simulink model "SR-to-MP_simulation_system"  (R2019a)
settings: Solver=VariableStepAuto  StartTime=0.0  StopTime=720000  RelTol=1e-3
undefined symbols (not defined in the file or in its folder): des
settings Model: Creator=86180  LastModifiedBy=86180

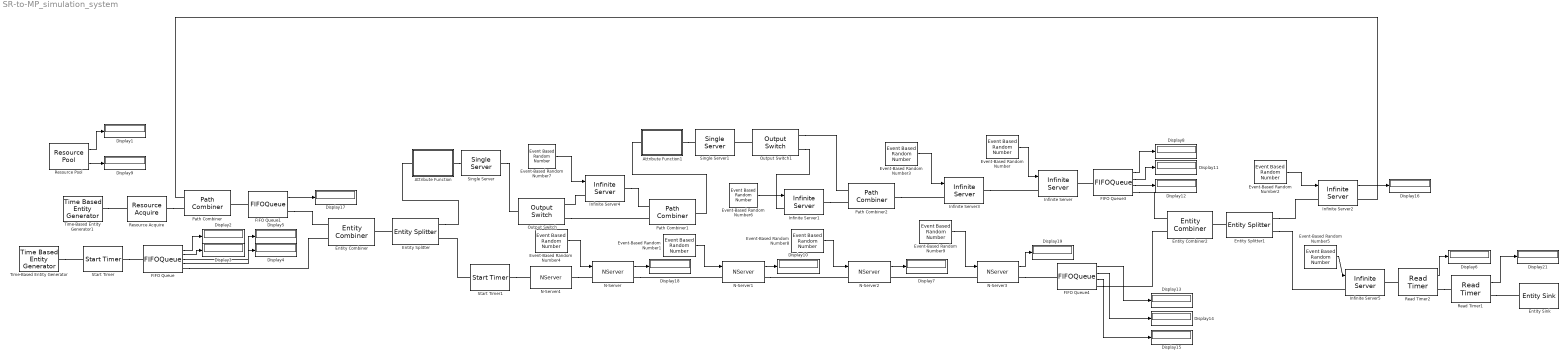
== system SR-to-MP_simulation_system ==
  Attribute Function : Subsystem  LoadFcn=des.afb.attributefunction_support(gcb,'LoadFcn');  StartFcn=des.afb.attributefunction_support(gcb,'StartFcn');  mask(Attribute Function){OutputNamePrefix=out_}
      mask prompts: OutputNamePrefix "Prefix name"
      settings: CopyFcn=des.afb.attributefunction_support(gcb,'CopyFcn');  OpenFcn=des.afb.attributefunction_support(gcb,'OpenFcn');  ErrorFcn=des.afb.error_redirect
      mask Help: slhelp(gcbh)
      mask Display: image(des_iconLoad('attribFunction.jpg'),'center');
  Attribute Function1 : Subsystem  LoadFcn=des.afb.attributefunction_support(gcb,'LoadFcn');  StartFcn=des.afb.attributefunction_support(gcb,'StartFcn');  mask(Attribute Function){OutputNamePrefix=out_}
      mask prompts: OutputNamePrefix "Prefix name"
      settings: CopyFcn=des.afb.attributefunction_support(gcb,'CopyFcn');  OpenFcn=des.afb.attributefunction_support(gcb,'OpenFcn');  ErrorFcn=des.afb.error_redirect
      mask Help: slhelp(gcbh)
      mask Display: image(des_iconLoad('attribFunction.jpg'),'center');
  Display{1..19,21} (20 alike) : Display
  Entity Combiner : EntityCombiner  NumberInputPorts=2
  Entity Combiner2 : EntityCombiner  NumberInputPorts=2
  Entity Sink : EntitySink
  Entity Splitter : EntitySplitter  NumberOutputPorts=2
  Entity Splitter1 : EntitySplitter  NumberOutputPorts=2
  Event-Based Random Number : EventBasedRandomNumber  meanExp=387  meanNorm=315  stdNorm=5  Seed=34425
  Event-Based Random Number1 : EventBasedRandomNumber  meanExp=234  meanNorm=7  stdNorm=38  Seed=3080
  Event-Based Random Number2 : EventBasedRandomNumber  meanExp=10  Seed=58140
  Event-Based Random Number3 : EventBasedRandomNumber  meanExp=10  meanNorm=12  stdNorm=3  Seed=11223
  Event-Based Random Number4 : EventBasedRandomNumber  meanExp=234  meanNorm=7  stdNorm=38  Seed=343
  Event-Based Random Number5 : EventBasedRandomNumber  meanExp=10  Seed=61357
  Event-Based Random Number6 : EventBasedRandomNumber  meanExp=3  meanNorm=12  stdNorm=3  Seed=251
  Event-Based Random Number7 : EventBasedRandomNumber  meanExp=3  meanNorm=12  stdNorm=3  Seed=2512
  Event-Based Random Number8 : EventBasedRandomNumber  meanExp=234  meanNorm=7  stdNorm=38  Seed=3423
  Event-Based Random Number9 : EventBasedRandomNumber  meanExp=234  meanNorm=7  stdNorm=38  Seed=3423
  FIFO Queue : FIFOQueue  Capacity=10000  StatNumberDeparted=on  StatNumberInBlock=on  StatAverageWait=on  StatAverageQueueLength=on
      settings: OutputPortMap=o0,o1,o2,o3
  FIFO Queue1 : FIFOQueue  Capacity=100  StatAverageQueueLength=on
      settings: OutputPortMap=o3
  FIFO Queue3 : FIFOQueue  StatNumberDeparted=on  StatAverageWait=on  StatAverageQueueLength=on
      settings: OutputPortMap=o0,o2,o3
  FIFO Queue4 : FIFOQueue  Capacity=6  StatNumberDeparted=on  StatAverageWait=on  StatAverageQueueLength=on
      settings: OutputPortMap=o0,o2,o3
  Infinite Server{,1,3..5} (5 alike) : InfiniteServer  ServiceTimeFrom=Signal port t
  Infinite Server2 : InfiniteServer  ServiceTimeFrom=Signal port t  StatNumberDeparted=on
  N-Server{,1..3} (4 alike) : NServer  NumberOfServers=6  ServiceTimeFrom=Signal port t  StatUtilization=on
      settings: OutputPortMap=o5
  N-Server4 : NServer  NumberOfServers=10  ServiceTime=0
  Output Switch : OutputSwitch  NumberOutputPorts=2  SwitchingCriterion=From attribute  AttributeName=Attribute
  Output Switch1 : OutputSwitch  NumberOutputPorts=2  SwitchingCriterion=From attribute  AttributeName=Attribute2
  Path Combiner : PathCombiner  NumberInputPorts=2
  Path Combiner1 : PathCombiner  NumberInputPorts=2
  Path Combiner2 : PathCombiner  NumberInputPorts=2
  Read Timer1 : ReadTimer  TimerTag=T2  StatAverageTimeElapsed=on
      settings: OutputPortMap=o3
  Read Timer2 : ReadTimer  StatAverageTimeElapsed=on
      settings: OutputPortMap=o3
  Resource Acquire : ResourceAcquire  ResourceName=robot  Capacity=100  EvaluatedResourceAmount={ 1}
  Resource Pool : ResourcePool  ResourceName=robot  ResourceAmount=18  StatAmountInUse=on  StatUtilization=on
      settings: OutputPortMap=o0,o1
  Single Server : SingleServer  ServiceTime=0
  Single Server1 : SingleServer  ServiceTime=0
  Start Timer : StartTimer  TimerTag=T2  TimerStartedOption=Continue
  Start Timer1 : StartTimer  TimerStartedOption=Continue
  Time-Based Entity Generator : TimeBasedEntityGenerator  Distribution=Exponential  InitialSeed=40859  Mean=3600/60
  Time-Based Entity Generator1 : TimeBasedEntityGenerator  Period=0.00000001  Mean=3600/20
  wires:
  Event-Based Random Number1/1 -> N-Server1/1
  Event-Based Random Number4/1 -> N-Server/1
  Event-Based Random Number2/1 -> Infinite Server2/1
  FIFO Queue4/1 -> Display13/1
  FIFO Queue4/2 -> Display14/1
  Resource Pool/1 -> Display1/1
  Infinite Server2/1 -> Display16/1
  Event-Based Random Number/1 -> Infinite Server/1
  FIFO Queue/4 -> Display4/1
  Event-Based Random Number3/1 -> Infinite Server3/1
  FIFO Queue3/3 -> Display12/1
  FIFO Queue1/1 -> Display17/1
  FIFO Queue/3 -> Display5/1
  Read Timer1/1 -> Display21/1
  Event-Based Random Number5/1 -> Infinite Server5/1
  FIFO Queue4/3 -> Display15/1
  FIFO Queue3/1 -> Display8/1
  FIFO Queue/2 -> Display3/1
  Read Timer2/1 -> Display6/1
  FIFO Queue/1 -> Display2/1
  Resource Pool/2 -> Display9/1
  FIFO Queue3/2 -> Display11/1
  Event-Based Random Number6/1 -> Infinite Server1/1
  Event-Based Random Number7/1 -> Infinite Server4/1
  Event-Based Random Number8/1 -> N-Server2/1
  Event-Based Random Number9/1 -> N-Server3/1
  N-Server2/1 -> Display7/1
  N-Server1/1 -> Display10/1
  N-Server/1 -> Display18/1
  N-Server3/1 -> Display19/1
  connections:
  Entity Splitter1/RConn2 -- Infinite Server5/LConn1
  FIFO Queue3/LConn1 -- Infinite Server/RConn1
  N-Server/RConn1 -- N-Server1/LConn1
  Read Timer2/LConn1 -- Infinite Server5/RConn1
  Time-Based Entity Generator/RConn1 -- Start Timer/LConn1
  FIFO Queue/RConn1 -- Entity Combiner/LConn2
  Resource Acquire/RConn1 -- Path Combiner/LConn2
  Infinite Server3/RConn1 -- Infinite Server/LConn1
  Path Combiner/LConn1 -- Infinite Server2/RConn1
  Start Timer/RConn1 -- FIFO Queue/LConn1
  Entity Splitter/LConn1 -- Entity Combiner/RConn1
  Read Timer1/RConn1 -- Entity Sink/LConn1
  FIFO Queue1/RConn1 -- Entity Combiner/LConn1
  Entity Splitter1/LConn1 -- Entity Combiner2/RConn1
  FIFO Queue3/RConn1 -- Entity Combiner2/LConn1
  Time-Based Entity Generator1/RConn1 -- Resource Acquire/LConn1
  Read Timer2/RConn1 -- Read Timer1/LConn1
  Entity Splitter1/RConn1 -- Infinite Server2/LConn1
  Start Timer1/LConn1 -- Entity Splitter/RConn2
  FIFO Queue1/LConn1 -- Path Combiner/RConn1
  FIFO Queue4/RConn1 -- Entity Combiner2/LConn2
  Infinite Server4/LConn1 -- Output Switch/RConn1
  Entity Splitter/RConn1 -- Attribute Function/LConn1
  Output Switch/RConn2 -- Path Combiner1/LConn2
  Infinite Server1/RConn1 -- Path Combiner2/LConn2
  Path Combiner2/RConn1 -- Infinite Server3/LConn1
  N-Server1/RConn1 -- N-Server2/LConn1
  N-Server3/LConn1 -- N-Server2/RConn1
  N-Server3/RConn1 -- FIFO Queue4/LConn1
  Attribute Function/RConn1 -- Single Server/LConn1
  Single Server/RConn1 -- Output Switch/LConn1
  Attribute Function1/RConn1 -- Single Server1/LConn1
  Output Switch1/LConn1 -- Single Server1/RConn1
  Infinite Server4/RConn1 -- Path Combiner1/LConn1
  Attribute Function1/LConn1 -- Path Combiner1/RConn1
  Output Switch1/RConn1 -- Path Combiner2/LConn1
  Output Switch1/RConn2 -- Infinite Server1/LConn1
  Start Timer1/RConn1 -- N-Server4/LConn1
  N-Server4/RConn1 -- N-Server/LConn1

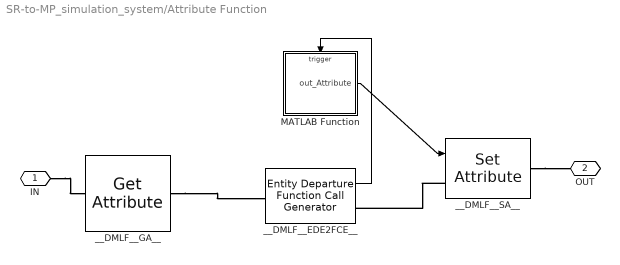
== system SR-to-MP_simulation_system/Attribute Function ==
  MATLAB Function : MATLAB Function  TreatAsAtomicUnit=on
  __DMLF__EDE2FCE__ : EntityDepartureFunctionCallGenerator  TimingFunctionCallF1=Before entity departure  IsInsideAFB=on
  __DMLF__GA__ : GetAttribute  EvaluatedDefaultAttributeValue={ }  IsInsideAFB=on
  __DMLF__SA__ : SetAttribute  AttributeName=Attribute  AttributeFrom=Signal port  EvaluatedAttributeValue={ []}  IsInsideAFB=on
  IN : PMIOPort  Side=Left
  OUT : PMIOPort  Port=2  Side=Right
  wires:
  __DMLF__EDE2FCE__/1 -> MATLAB Function/Trigger
  MATLAB Function/1(out_Attribute) -> __DMLF__SA__/1
  connections:
  __DMLF__SA__/LConn1 -- __DMLF__EDE2FCE__/RConn1
  __DMLF__GA__/RConn1 -- __DMLF__EDE2FCE__/LConn1
  IN/RConn1 -- __DMLF__GA__/LConn1
  __DMLF__SA__/RConn1 -- OUT/RConn1

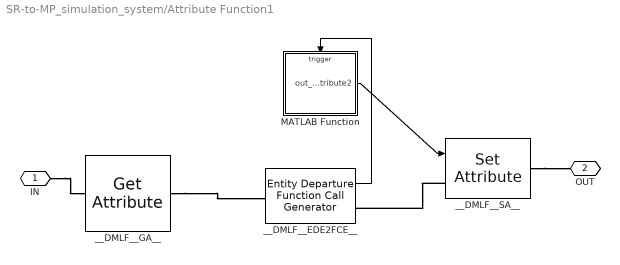
== system SR-to-MP_simulation_system/Attribute Function1 ==
  MATLAB Function : MATLAB Function  TreatAsAtomicUnit=on
  __DMLF__EDE2FCE__ : EntityDepartureFunctionCallGenerator  TimingFunctionCallF1=Before entity departure  IsInsideAFB=on
  __DMLF__GA__ : GetAttribute  EvaluatedDefaultAttributeValue={ }  IsInsideAFB=on
  __DMLF__SA__ : SetAttribute  AttributeName=Attribute2  AttributeFrom=Signal port  EvaluatedAttributeValue={ []}  IsInsideAFB=on
  IN : PMIOPort  Side=Left
  OUT : PMIOPort  Port=2  Side=Right
  wires:
  __DMLF__EDE2FCE__/1 -> MATLAB Function/Trigger
  MATLAB Function/1(out_Attribute2) -> __DMLF__SA__/1
  connections:
  __DMLF__SA__/LConn1 -- __DMLF__EDE2FCE__/RConn1
  __DMLF__GA__/RConn1 -- __DMLF__EDE2FCE__/LConn1
  IN/RConn1 -- __DMLF__GA__/LConn1
  __DMLF__SA__/RConn1 -- OUT/RConn1

== matlab function SR-to-MP_simulation_system/Attribute Function/MATLAB Function ==
  data: out_Attribute output
  events: trigger input FUNCTION_CALL_EVENT
function out_Attribute = fcn()
%FCN    Access and modify attributes with MATLAB 
% 
% Input arguments must match the attribute names.
% Output arguments must be out_<AttributeName>,
% e.g., out_ServiceTime where ServiceTime is the attribute name.
% 
% The output attribute will be created if it is not present.
%

x = rand();
if x<= 0.5
    out_Attribute = 1;
else
    out_Attribute = 2;
end

== matlab function SR-to-MP_simulation_system/Attribute Function1/MATLAB Function ==
  data: out_Attribute2 output
  events: trigger input FUNCTION_CALL_EVENT
function out_Attribute2 = fcn()
%FCN    Access and modify attributes with MATLAB 
% 
% Input arguments must match the attribute names.
% Output arguments must be out_<AttributeName>,
% e.g., out_ServiceTime where ServiceTime is the attribute name.
% 
% The output attribute will be created if it is not present.
%

x = rand();
if x<= 0.5
    out_Attribute2 = 1;
else
    out_Attribute2 = 2;
end
